simulink model "baseModel"  (R2021b)
settings: Solver=VariableStepAuto  StartTime=0.0  StopTime=10.0  RelTol=1e-3
values from neighbouring files (symbols this model uses):
  dt = 0.004    [main.m]    (also in runModel.m = 0.001)
undefined symbols (not defined in the file or in its folder): droneParams, modelParams, state
libraries: uavutilslib x1
settings Model: Creator=jbeers  LastModifiedBy=jbeers

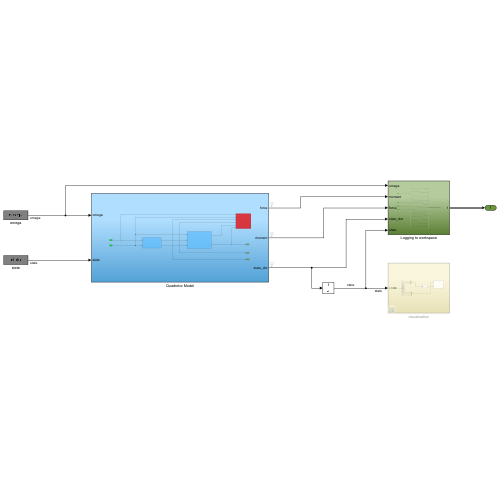
[thumbnail: Simulink's stored preview of the top-level diagram]
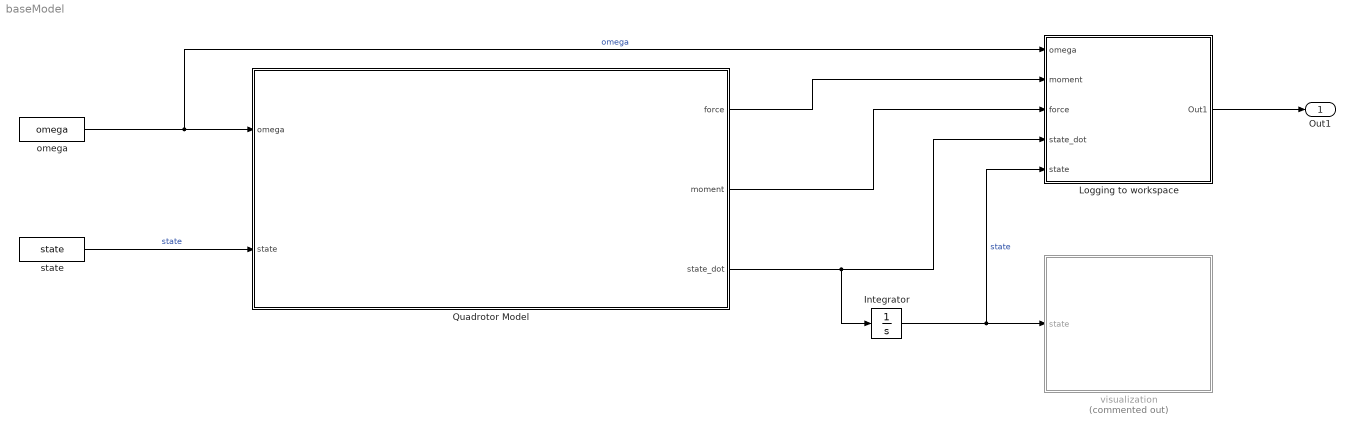
== system baseModel ==
  Integrator : Integrator  InitialCondition=state.signals.values(1, :)
  Logging to workspace : Subsystem
  Quadrotor Model : Subsystem
  omega : FromWorkspace  VariableName=omega  SampleTime=dt
  state : FromWorkspace  VariableName=state
  visualization : Subsystem  Commented=on
  Out1 : Outport
  wires:
  Quadrotor Model/1(force) -> Logging to workspace/2(moment)
  omega/1 -> Logging to workspace/1(omega), Quadrotor Model/1(omega)  "omega"
  Quadrotor Model/2(moment) -> Logging to workspace/3(force)
  Integrator/1 -> visualization/1(state), Logging to workspace/5(state)  "state"
  Logging to workspace/1(Out1) -> Out1/1
  Quadrotor Model/3(state_dot) -> Logging to workspace/4(state_dot), Integrator/1
  state/1 -> Quadrotor Model/2(state)  "state"

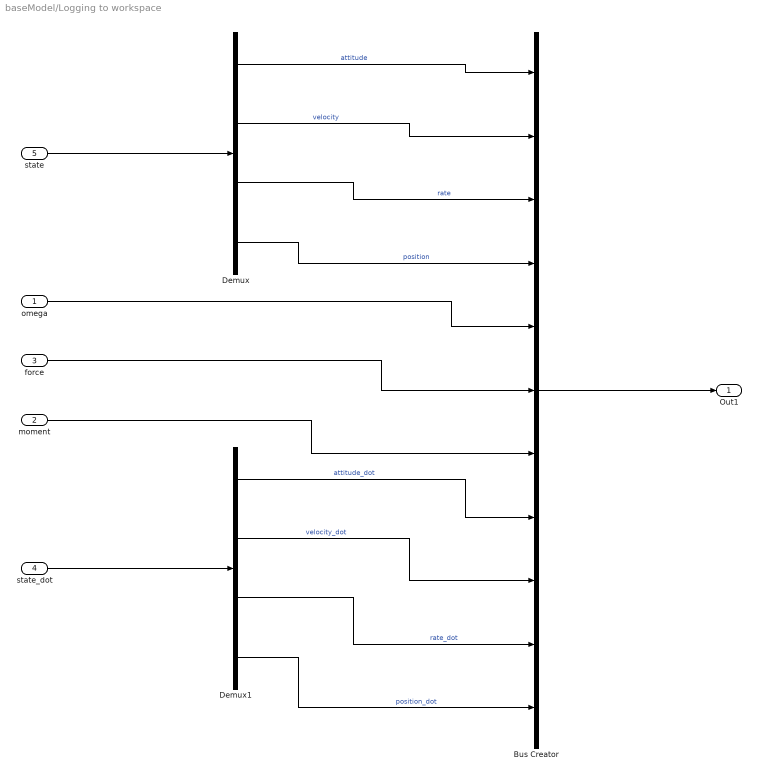
== system baseModel/Logging to workspace ==
  omega : Inport
  moment : Inport  Port=2
  force : Inport  Port=3
  state_dot : Inport  Port=4
  state : Inport  Port=5
  Bus Creator : BusCreator  Inputs=11
  Demux : Demux
  Demux1 : Demux
  Out1 : Outport
  wires:
  omega/1 -> Bus Creator/5
  Demux/4 -> Bus Creator/4  "position"
  Demux/1 -> Bus Creator/1  "attitude"
  Demux/3 -> Bus Creator/3  "rate"
  Demux/2 -> Bus Creator/2  "velocity"
  state/1 -> Demux/1
  force/1 -> Bus Creator/6
  moment/1 -> Bus Creator/7
  Demux1/4 -> Bus Creator/11  "position_dot"
  state_dot/1 -> Demux1/1
  Demux1/2 -> Bus Creator/9  "velocity_dot"
  Demux1/1 -> Bus Creator/8  "attitude_dot"
  Demux1/3 -> Bus Creator/10  "rate_dot"
  Bus Creator/1 -> Out1/1

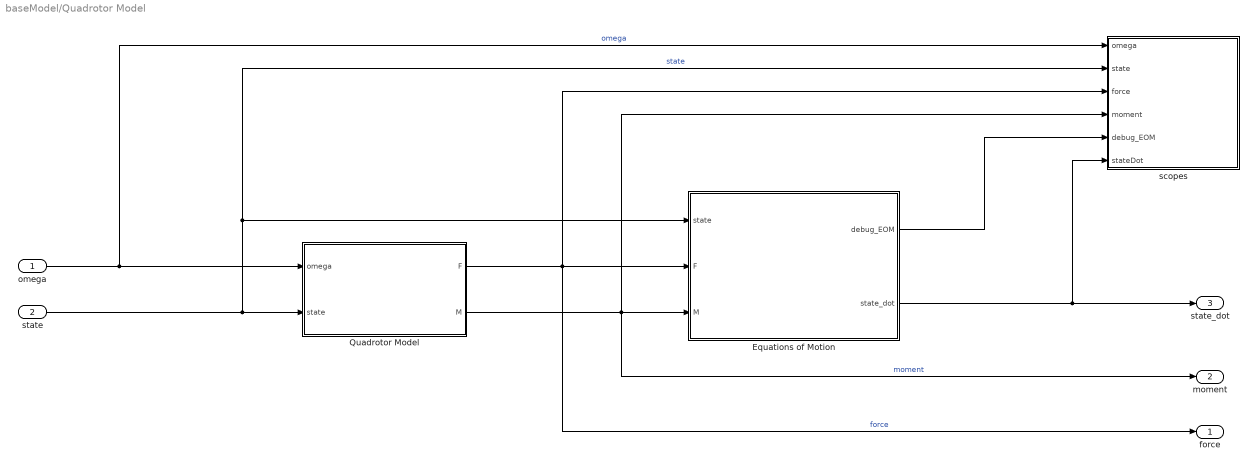
== system baseModel/Quadrotor Model ==
  omega : Inport  OutMin=droneParams.minRPM  OutMax=droneParams.maxRPM  PortDimensions=4
  state : Inport  Port=2  PortDimensions=12
  Equations of Motion : MATLAB Function  TreatAsAtomicUnit=on
  Quadrotor Model : MATLAB Function  TreatAsAtomicUnit=on
  scopes : Subsystem
  force : Outport  PortDimensions=3
  moment : Outport  Port=2  PortDimensions=3
  state_dot : Outport  Port=3  PortDimensions=12
  wires:
  state/1 -> scopes/2(state), Equations of Motion/1(state), Quadrotor Model/2(state)  "state"
  Quadrotor Model/2(M) -> moment/1, scopes/4(moment), Equations of Motion/3(M)  "moment"
  Equations of Motion/2(state_dot) -> scopes/6(stateDot), state_dot/1
  omega/1 -> Quadrotor Model/1(omega), scopes/1(omega)  "omega"
  Quadrotor Model/1(F) -> force/1, Equations of Motion/2(F), scopes/3(force)  "force"
  Equations of Motion/1(debug_EOM) -> scopes/5(debug_EOM)

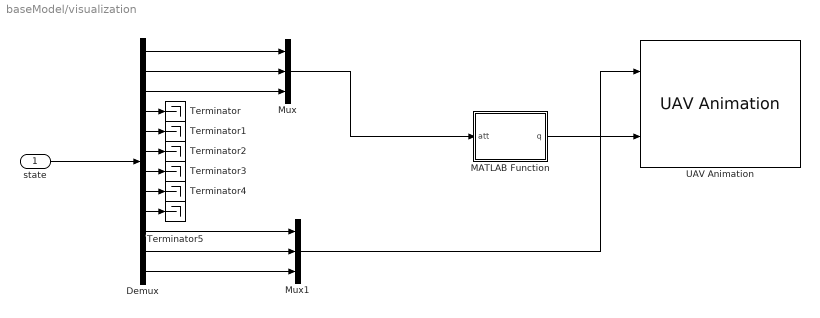
== system baseModel/visualization ==
  state : Inport
  Demux : Demux  Outputs=12
  MATLAB Function : MATLAB Function  TreatAsAtomicUnit=on
  Mux : Mux  Inputs=3
  Mux1 : Mux  Inputs=3
  Terminator{,1..5} (6 alike) : Terminator
  UAV Animation : uavutilslib/UAV Animation  UAVType=Multirotor  UAVSize=2*droneParams.b  InertialZDirection=Down  SampleTime=-1
      settings: SourceProductBaseCode=UV
  wires:
  Mux1/1 -> UAV Animation/1
  Demux/3 -> Mux/3
  Demux/2 -> Mux/2
  Demux/4 -> Terminator/1
  Mux/1 -> MATLAB Function/1(att)
  Demux/11 -> Mux1/2
  Demux/12 -> Mux1/3
  Demux/1 -> Mux/1
  Demux/10 -> Mux1/1
  MATLAB Function/1(q) -> UAV Animation/2
  Demux/5 -> Terminator1/1
  state/1 -> Demux/1
  Demux/7 -> Terminator3/1
  Demux/9 -> Terminator5/1
  Demux/8 -> Terminator4/1
  Demux/6 -> Terminator2/1

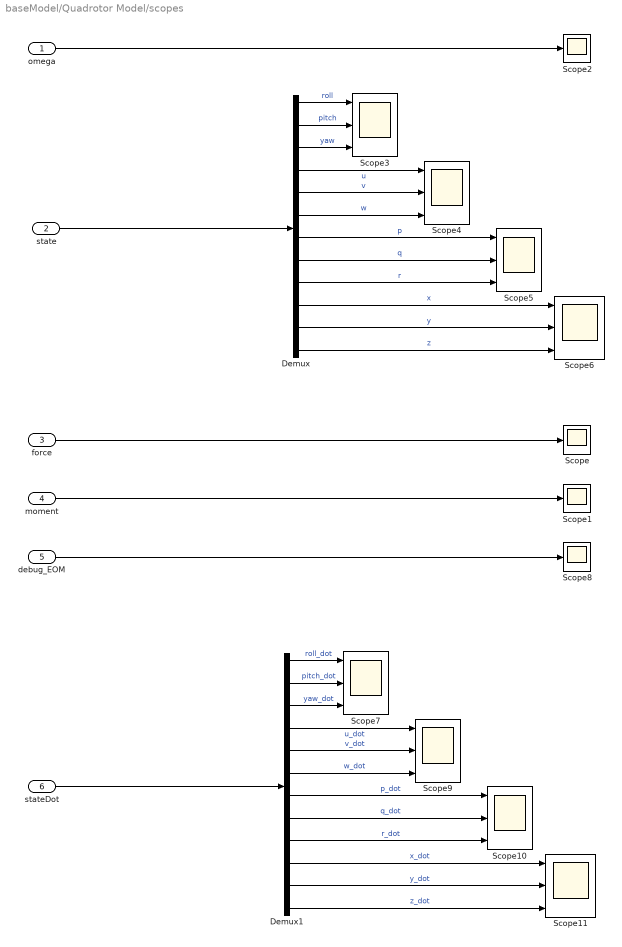
== system baseModel/Quadrotor Model/scopes ==
  omega : Inport
  state : Inport  Port=2
  force : Inport  Port=3
  moment : Inport  Port=4
  debug_EOM : Inport  Port=5
  stateDot : Inport  Port=6
  Demux : Demux  Outputs=12
  Demux1 : Demux  Outputs=12
  Scope{,1..2,8} (4 alike) : Scope
  Scope{3..7,9..11} (8 alike) : Scope  NumInputPorts=3
  wires:
  Demux/12 -> Scope6/3  "z"
  Demux/7 -> Scope5/1  "p"
  Demux/8 -> Scope5/2  "q"
  Demux/1 -> Scope3/1  "roll"
  Demux/2 -> Scope3/2  "pitch"
  Demux/5 -> Scope4/2  "v"
  Demux/11 -> Scope6/2  "y"
  Demux/10 -> Scope6/1  "x"
  Demux/3 -> Scope3/3  "yaw"
  omega/1 -> Scope2/1
  Demux/9 -> Scope5/3  "r"
  Demux/4 -> Scope4/1  "u"
  Demux/6 -> Scope4/3  "w"
  state/1 -> Demux/1
  debug_EOM/1 -> Scope8/1
  force/1 -> Scope/1
  moment/1 -> Scope1/1
  Demux1/3 -> Scope7/3  "yaw_dot"
  stateDot/1 -> Demux1/1
  Demux1/6 -> Scope9/3  "w_dot"
  Demux1/4 -> Scope9/1  "u_dot"
  Demux1/9 -> Scope10/3  "r_dot"
  Demux1/10 -> Scope11/1  "x_dot"
  Demux1/5 -> Scope9/2  "v_dot"
  Demux1/2 -> Scope7/2  "pitch_dot"
  Demux1/11 -> Scope11/2  "y_dot"
  Demux1/1 -> Scope7/1  "roll_dot"
  Demux1/12 -> Scope11/3  "z_dot"
  Demux1/8 -> Scope10/2  "q_dot"
  Demux1/7 -> Scope10/1  "p_dot"

== matlab function baseModel/Quadrotor Model/Equations of Motion ==
  data: debug_EOM output; state input; F input; state_dot output; M input; droneParams parameter; modelParams parameter
% function state_dot = EOM(state, F, M, droneParams, modelParams)
function [debug_EOM, state_dot] = EOM(state, F, M, droneParams, modelParams)
    % Function to compute the quadrotor equations of motion
    % state = [roll, pitch, yaw, u, v, w, p, q, r, x, y, z]
    %   - Attitude: [roll, pitch, yaw] in rad
    %   - (Body) velocity: [u, v, w] in m/s
    %   - (Body) rotational rates: [p, q, r] in rad/s
    %   - Position: [x, y, z] in E-frame, in m

    % Extract necessary drone parameters
    mass = droneParams.mass;
    Iv = droneParams.Iv;
    invIv = inv(Iv);
    g = modelParams.g;
    gVec = [0; 0; g];

    % Pre-allocate state derivative array
    state_dot = zeros(size(state));

    % Compute accelerations
    linAcc = (F/mass)' + QuatRot(gVec, state(1:3), "E2B") - cross(state(7:9), state(4:6));
    rotAcc = invIv*M' - invIv * (cross(state(7:9), Iv*state(7:9)));

    % Fill in state derivative
    state_dot(1:3) = PQR_to_AttDot_Euler(state(1:3), state(7:9));
    state_dot(4:6) = linAcc;
    state_dot(7:9) = rotAcc;
    state_dot(10:12) = QuatRot(state(4:6), state(1:3), "B2E");

    % Debugging
    debug_EOM = 0;

== matlab function baseModel/Quadrotor Model/Quadrotor Model ==
  data: omega input; state input; F output; M output; droneParams parameter; modelParams parameter
function [F, M] = getForcesMoments(omega, state, droneParams, modelParams)
    % Call function getFM() from workspace
    [F, M] = getFM(state, omega, modelParams, droneParams);

== matlab function baseModel/visualization/MATLAB Function ==
  data: att input; q output
function q = E2Q(att)

q = Eul2Quat(att);
